simulink model "matprob1"  (R2020a)
settings: Solver=VariableStepAuto  StartTime=0.0  StopTime=10.0  RelTol=1e-3
values from neighbouring files (symbols this model uses):
  b1 = 50    [matprob1.mat]
  k1 = 50    [matprob1.mat]
  k2 = 25    [matprob1.mat]
  m1 = 100    [matprob1.mat]
  m2 = 50    [matprob1.mat]
settings Model: Creator=deepa  LastModifiedBy=deepa

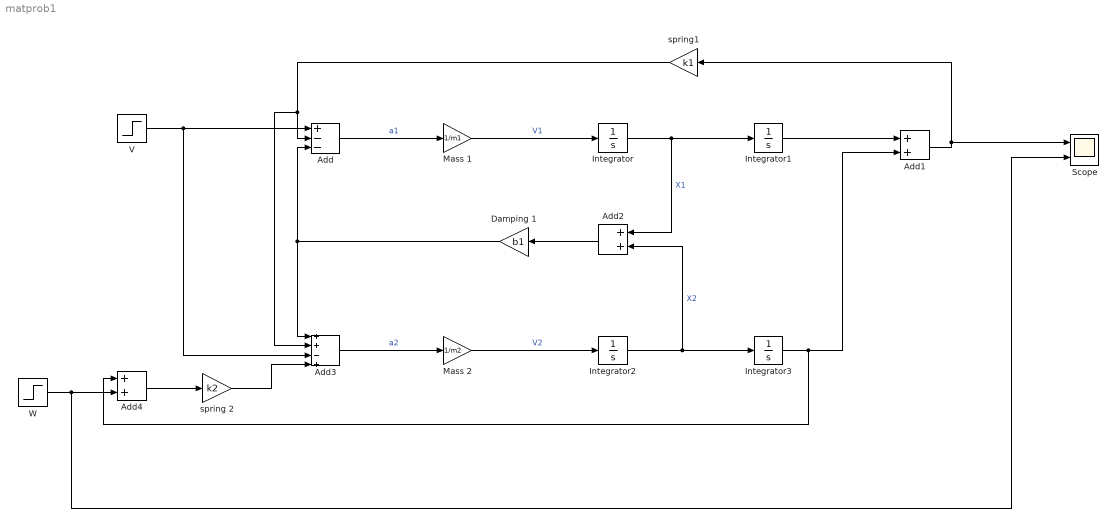
== system matprob1 ==
  Add : Sum  Inputs=+--
  Add1 : Sum
  Add2 : Sum
  Add3 : Sum  Inputs=++-+
  Add4 : Sum
  Damping 1 : Gain  Gain=b1
  Integrator{,1..3} (4 alike) : Integrator
  Mass 1 : Gain  Gain=1/m1
  Mass 2 : Gain  Gain=1/m2
  Scope : Scope  NumInputPorts=2
  V : Step  SampleTime=0
  W : Step  SampleTime=0
  spring 2 : Gain  Gain=k2
  spring1 : Gain  Gain=k1
  wires:
  Add/1 -> Mass 1/1  "a1"
  Mass 1/1 -> Integrator/1  "V1"
  Integrator/1 -> Add2/1, Integrator1/1  "X1"
  Integrator1/1 -> Add1/1
  Add1/1 -> spring1/1, Scope/1
  spring1/1 -> Add3/2, Add/2
  Damping 1/1 -> Add3/1, Add/3
  Add2/1 -> Damping 1/1
  Add3/1 -> Mass 2/1  "a2"
  Mass 2/1 -> Integrator2/1  "V2"
  Integrator2/1 -> Add2/2, Integrator3/1  "X2"
  Integrator3/1 -> Add4/1, Add1/2
  V/1 -> Add/1, Add3/3
  spring 2/1 -> Add3/4
  Add4/1 -> spring 2/1
  W/1 -> Scope/2, Add4/2
